simulink model "coord_test2"  (R2013a)
settings: Solver=ode45  StartTime=0.0  StopTime=10.0  RelTol=1e-3
libraries: QuaternionLib x4
settings Model: Creator=EwingKang  LastModifiedBy=EwingKang

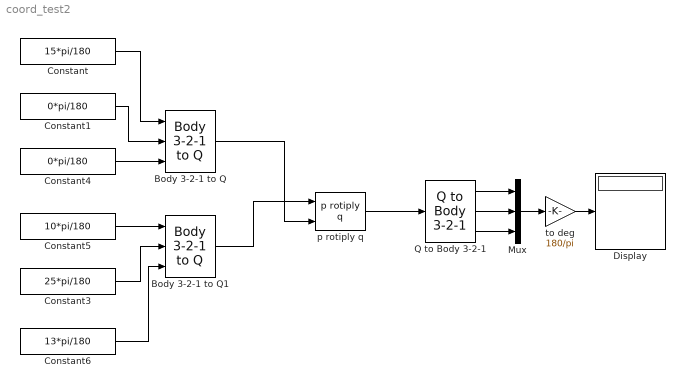
== system coord_test2 ==
  Body 3-2-1 to Q : QuaternionLib/Body 3-2-1 to Q
  Body 3-2-1 to Q1 : QuaternionLib/Body 3-2-1 to Q
  Constant : Constant  Value=15*pi/180
  Constant1 : Constant  Value=0*pi/180
  Constant3 : Constant  Value=25*pi/180
  Constant4 : Constant  Value=0*pi/180
  Constant5 : Constant  Value=10*pi/180
  Constant6 : Constant  Value=13*pi/180
  Display : Display
  Mux : Mux  Inputs=3
  Q to Body 3-2-1 : QuaternionLib/Q to Body 3-2-1
  p rotiply q : QuaternionLib/p rotiply q
  to deg : Gain  Gain=180/pi
  wires:
  p rotiply q/1 -> Q to Body 3-2-1/1
  Mux/1 -> to deg/1
  Q to Body 3-2-1/2 -> Mux/2
  Q to Body 3-2-1/1 -> Mux/1
  Q to Body 3-2-1/3 -> Mux/3
  to deg/1 -> Display/1
  Body 3-2-1 to Q/1 -> p rotiply q/2
  Body 3-2-1 to Q1/1 -> p rotiply q/1
  Constant5/1 -> Body 3-2-1 to Q1/1
  Constant3/1 -> Body 3-2-1 to Q1/2
  Constant6/1 -> Body 3-2-1 to Q1/3
  Constant/1 -> Body 3-2-1 to Q/1
  Constant1/1 -> Body 3-2-1 to Q/2
  Constant4/1 -> Body 3-2-1 to Q/3
